simulink model "fdgdf"  (R2020b)
settings: Solver=VariableStepAuto  StartTime=0.0  StopTime=10.0  RelTol=1e-3
values from neighbouring files (symbols this model uses):
  A = [0 1 0 0 0 0; 0 0 1 0 0 0; 0 0 0 1 0 0; 0 0 -k/m -b/m 0 0; 0 0 0 0 0 1; 0 0 0 0 0 0]    [accel_jerk_ctrl_testbed.m]    (also in halfcarsuspensionlinearization.m = double(subs(J_a, {x1 x2 x3 x4 x5 x6 x7 x8 zrr zrf fr ff},[0,; quartersuspensionscript.m = [ 0 1 0 0; [-k_spring -b_damper k_spring b_damper]/m_car ; 0)
  B = [0 0 0 k/m 0 1]'    [accel_jerk_ctrl_testbed.m]    (also in halfcarsuspensionlinearization.m = double(subs(J_b, {x1 x2 x3 x4 x5 x6 x7 x8 zrr zrf fr ff},[0,; quartersuspensionscript.m = [ 0; 0; 0; k_wheel/m_wheel])
  C = eye(8)    [halfcarsuspensionlinearization.m]
  D = zeros(8,2)    [halfcarsuspensionlinearization.m]
  KK = lqr(sys,eye(8),.00000001*eye(2))    [halfcarsuspensionlinearization.m]
undefined symbols (not defined in the file or in its folder): Continuous, Time
libraries: simulink x1, ctrlSharedLib x1, cstblocks x1
settings Model: Creator=Ricky  LastModifiedBy=Ricky

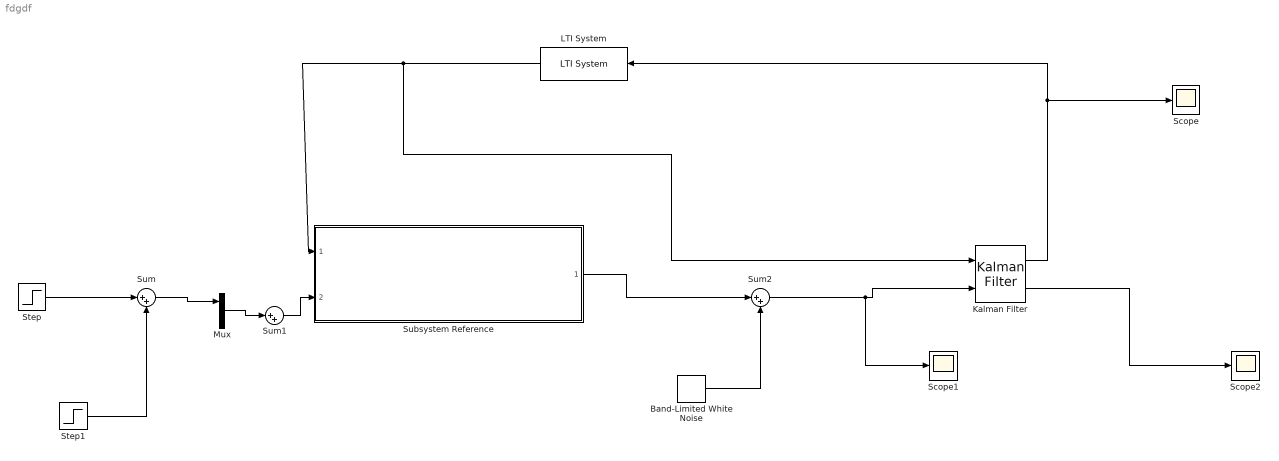
== system fdgdf ==
  Band-Limited White Noise : simulink/Sources/Band-Limited White Noise  Cov=[0.001]  Ts=0.1  seed=[23341]
  Kalman Filter : ctrlSharedLib/Kalman Filter  TimeDomain=Continuous-Time  UseCurrentEstimator=on  ModelSource=Individual A, B, C, D matrices  ModelSourceVariable=ss(0.95,1,1,0,1)  A=A  B=B  C=C  D=D  NumberOfStates=1  NumberOfInputs=1  NumberOfOutputs=1  InitialEstimateSource=Dialog  X0=0  P0=10  UseK=off  UseGH=off  NumberOfProcessNoiseInputs=1  G=1  TimeInvariantG=on  H=0  TimeInvariantH=on  Q=0.05  TimeInvariantQ=on  R=1  TimeInvariantR=on  N=0  TimeInvariantN=on  AddInputPort=on  AddEnablePort=off  OutputEstimatedY=on  OutputP=off  Ts=-1
  LTI System : cstblocks/LTI System  sys=-1*KK  IC=[]
  Mux : Mux  Inputs=2
  Scope : Scope
  Scope1 : Scope
  Scope2 : Scope
  Step : Step  After=.1  SampleTime=0
  Step1 : Step  Time=2  After=-.1  SampleTime=0
  Subsystem Reference : Subsystem  ReferencedSubsystem=halfcar_subsystem
  Sum : Sum  Inputs=|++
  Sum1 : Sum  Inputs=|++
  Sum2 : Sum  Inputs=|++
  wires:
  Step/1 -> Sum/1
  Step1/1 -> Sum/2
  Sum/1 -> Mux/1
  Mux/1 -> Sum1/1
  Sum1/1 -> Subsystem Reference/2
  Kalman Filter/1 -> LTI System/1, Scope/1
  LTI System/1 -> Kalman Filter/1, Subsystem Reference/1
  Sum2/1 -> Scope1/1, Kalman Filter/2
  Subsystem Reference/1 -> Sum2/1
  Band-Limited White Noise/1 -> Sum2/2
  Kalman Filter/2 -> Scope2/1
